simulink model "Vbyf_OpenLoop_Frequencycontrol"  (R2023a)
settings: Solver=FixedStepAuto  StartTime=0.0  StopTime=10.0  FixedStep=1e-6  RelTol=1e-3
libraries: spsIGBTDiodeLib x6, spsCurrentMeasurementLib x3, spsAsynchronousMachineSIUnitsLib x1, simulink x1, spsDCVoltageSourceLib x1, sps_lib x1
settings Model: Creator=hsriv  LastModifiedBy=hsriv

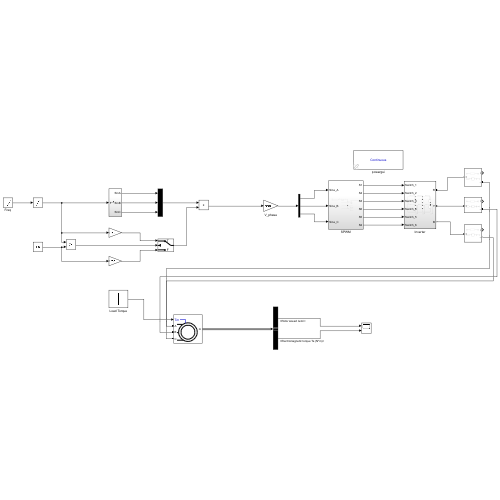
[thumbnail: Simulink's stored preview of the top-level diagram]
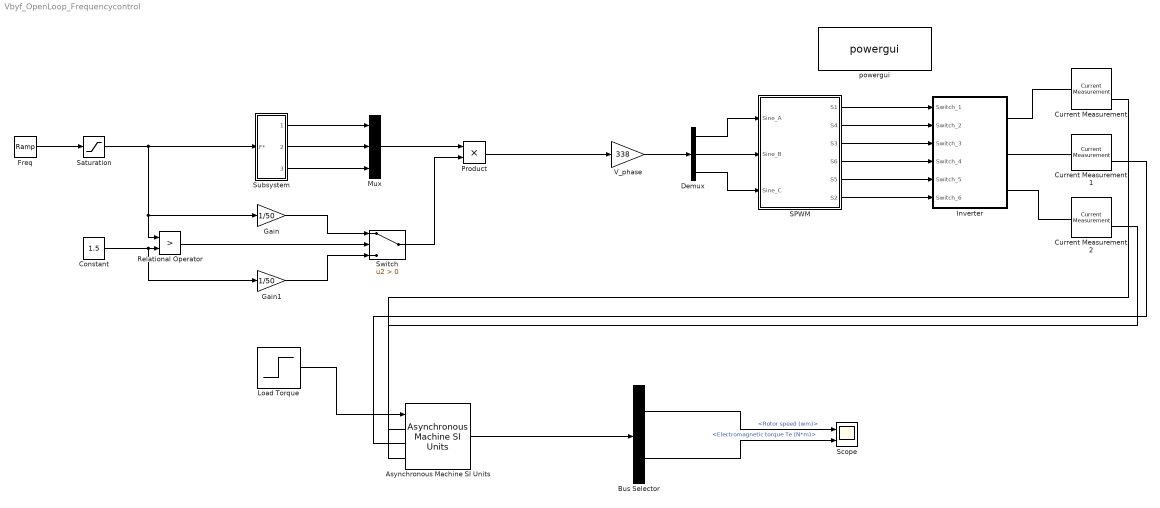
== system Vbyf_OpenLoop_Frequencycontrol ==
  Asynchronous Machine SI Units : spsAsynchronousMachineSIUnitsLib/Asynchronous Machine SI Units  RotorType=Squirrel-cage  PresetModel=No  MechanicalLoad=Torque Tm  ShowDetailedParameters=on  ReferenceFrame=Rotor  Units=SI  MeasurementBus=off  NominalParameters=[1.845e+04 415 50]  VoltageRatio=1  Stator=[0.5968 0.0003495]  Rotor=[0.6258 0.005473]  Cage1=[0.4155 0.002066]  Cage2=[0.4168 0.0003495]  Lm=0.0354  Mechanical=[0.05 0.005879 2]  PolePairs=2  InitialConditions=[1 0 0 0 0 0 0 0]  SimulateSaturation=off  Saturation=[14.03593122, 27.81365428, 53.79336849, 72.68890987, 97.98006896, 148.6815601, 215.7428561, 302.9841135, 428.7778367 ; 230, 322, 414, 460, 506, 552, 598, 644, 690]  LoadFlowParameters=1492000  TsPowergui=0  TsBlock=-1  IterativeModel=Trapezoidal non iterative  IterativeDiscreteModel=Trapezoidal non iterative  Pmec=1.492e+006
  Bus Selector : BusSelector  OutputSignals=Mechanical.Rotor speed (wm),Mechanical.Electromagnetic torque Te (N*m)
  Constant : Constant  Value=1.5
  Current Measurement : spsCurrentMeasurementLib/Current Measurement  PhasorSimulation=off  OutputType=Complex  PSBequivalent=0
  Current Measurement1 : spsCurrentMeasurementLib/Current Measurement  PhasorSimulation=off  OutputType=Complex  PSBequivalent=0
  Current Measurement2 : spsCurrentMeasurementLib/Current Measurement  PhasorSimulation=off  OutputType=Complex  PSBequivalent=0
  Demux : Demux  Outputs=3
  Freq : simulink/Sources/Ramp  slope=100  start=0  InitialOutput=0
  Gain : Gain  Gain=1/50
  Gain1 : Gain  Gain=1/50
  Inverter : Subsystem
  Load Torque : Step  Time=10  Before=0.00001  SampleTime=0
  Mux : Mux  Inputs=3
  Product : Product
  Relational Operator : RelationalOperator  Operator=>  OutDataTypeStr=boolean  RndMeth=Simplest  InputSameDT=off
  SPWM : Subsystem
  Saturation : Saturate  UpperLimit=50  LowerLimit=0
  Scope : Scope  NumInputPorts=2
  Subsystem : Subsystem
  Switch : Switch  Criteria=u2 > Threshold  SaturateOnIntegerOverflow=off  InputSameDT=off
  V_phase : Gain  Gain=338
  powergui : sps_lib/powergui  Priority=1  SimulationMode=Continuous  SampleTime=50e-6  frequency=60  Iterations=50  frequencyindice=50  Pbase=100e6  ErrMax=1e-4  UnitsV=kV  UnitsW=MW  buscounter=0  FunctionMessages=off  echomessages=off  EnableUseOfTLC=off  CurrentSourceSwitches=off  DisableSnubberDevices=off  DisableRonSwitches=off  DisableVfSwitches=off  DisplayEquations=off  AutomaticDiscreteSolvers=off  SolverType=Tustin/Backward Euler (TBE)  Interpol=off  ExternalGateDelay=off  methode=off  Ts=100  x0status=blocks  SPID=on  SwTol=0  HookPort=off  NonlinearTolerance=1e-4  nMaxIteration=100  ContinueOnMaxIteration=off  RestoreLinks=warning  ResistiveCurrentMeasurement=off  Frange=[0:2:500]  Ylog=off  Xlog=on  ShowGrid=off  save=off  variable=ZData  structure=0  ZoomFFT=off  StartTime=0.0  cycles=1  DisplayStyle=1  fundamental=60  FreqAxis=off  MaxFrequency=1000  frequencyindicesteady=1  RmsSteady=1  display=off
  wires:
  Subsystem/1(SinA) -> Mux/1
  Saturation/1 -> Subsystem/1(F*), Gain/1, Relational Operator/1
  Gain/1 -> Switch/1
  Constant/1 -> Gain1/1, Relational Operator/2
  Subsystem/3(SinC) -> Mux/3
  Switch/1 -> Product/2
  Mux/1 -> Product/1
  Freq/1 -> Saturation/1
  Subsystem/2(SinB) -> Mux/2
  Gain1/1 -> Switch/3
  Relational Operator/1 -> Switch/2
  Product/1 -> V_phase/1
  V_phase/1 -> Demux/1
  Demux/2 -> SPWM/2(Sine_B)
  Demux/1 -> SPWM/1(Sine_A)
  Demux/3 -> SPWM/3(Sine_C)
  SPWM/1(S1) -> Inverter/1(Switch_1)
  SPWM/2(S4) -> Inverter/2(Switch_2)
  SPWM/3(S3) -> Inverter/3(Switch_3)
  SPWM/4(S6) -> Inverter/4(Switch_4)
  SPWM/5(S5) -> Inverter/5(Switch_5)
  SPWM/6(S2) -> Inverter/6(Switch_6)
  Asynchronous Machine SI Units/1 -> Bus Selector/1
  Load Torque/1 -> Asynchronous Machine SI Units/1
  Bus Selector/1 -> Scope/1  "<Rotor speed (wm)>"
  Bus Selector/2 -> Scope/2  "<Electromagnetic torque Te (N*m)>"
  connections:
  Inverter/RConn1 -- Current Measurement/LConn1
  Inverter/RConn2 -- Current Measurement1/LConn1
  Inverter/RConn3 -- Current Measurement2/LConn1
  Current Measurement/RConn1 -- Asynchronous Machine SI Units/LConn1
  Current Measurement1/RConn1 -- Asynchronous Machine SI Units/LConn2
  Asynchronous Machine SI Units/LConn3 -- Current Measurement2/RConn1

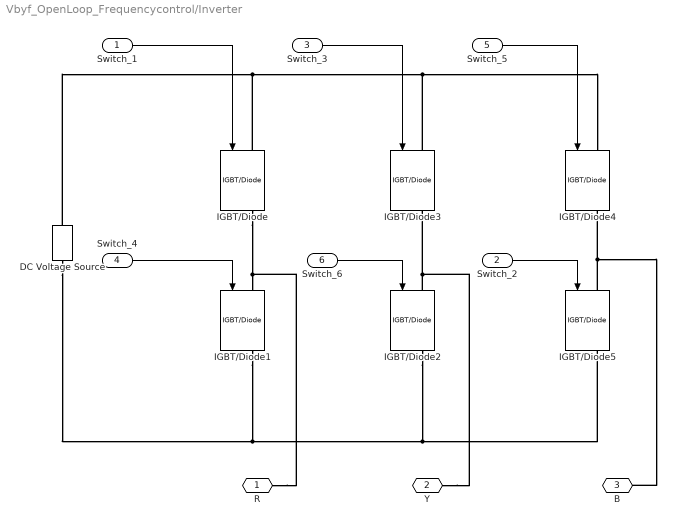
== system Vbyf_OpenLoop_Frequencycontrol/Inverter ==
  Switch_1 : Inport
  Switch_2 : Inport  Port=2
  Switch_3 : Inport  Port=3
  Switch_4 : Inport  Port=4
  Switch_5 : Inport  Port=5
  Switch_6 : Inport  Port=6
  DC Voltage Source : spsDCVoltageSourceLib/DC Voltage Source  Amplitude=700  Measurements=None
  IGBT/Diode{,1..5} (6 alike) : spsIGBTDiodeLib/IGBT//Diode  Ron=1e-3  Rs=1e5  Cs=inf  Measurements=on
  R : PMIOPort  Side=Right
  Y : PMIOPort  Port=2  Side=Right
  B : PMIOPort  Port=3  Side=Right
  wires:
  Switch_3/1 -> IGBT/Diode3/1
  Switch_6/1 -> IGBT/Diode2/1
  Switch_5/1 -> IGBT/Diode4/1
  Switch_4/1 -> IGBT/Diode1/1
  Switch_1/1 -> IGBT/Diode/1
  Switch_2/1 -> IGBT/Diode5/1
  connections:
  DC Voltage Source/LConn1 -- IGBT/Diode1/RConn1 -- IGBT/Diode5/RConn1 -- IGBT/Diode2/RConn1
  IGBT/Diode2/LConn1 -- IGBT/Diode3/RConn1 -- Y/RConn1
  DC Voltage Source/RConn1 -- IGBT/Diode3/LConn1 -- IGBT/Diode4/LConn1 -- IGBT/Diode/LConn1
  IGBT/Diode5/LConn1 -- B/RConn1 -- IGBT/Diode4/RConn1
  IGBT/Diode/RConn1 -- R/RConn1 -- IGBT/Diode1/LConn1

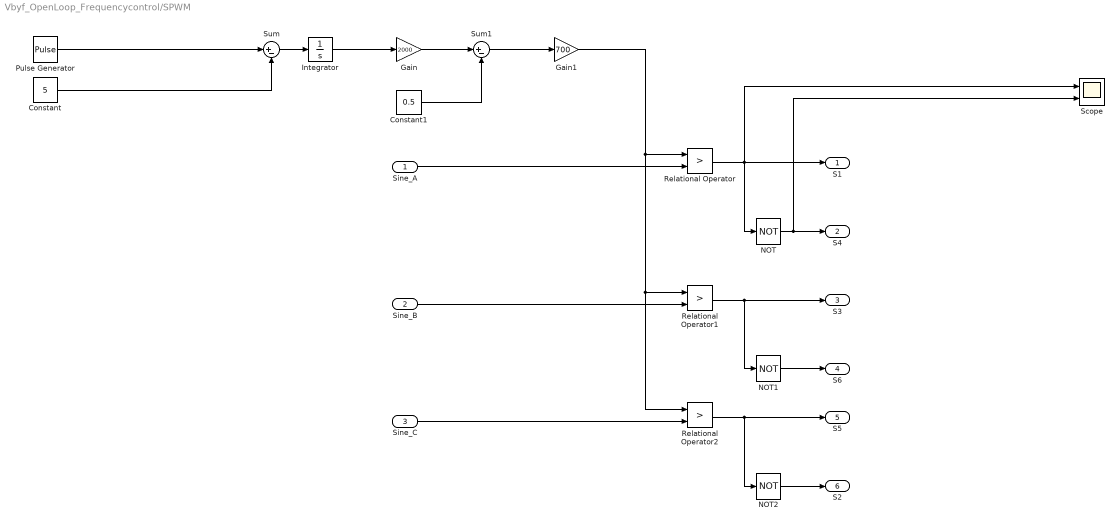
== system Vbyf_OpenLoop_Frequencycontrol/SPWM ==
  Sine_A : Inport
  Sine_B : Inport  Port=2
  Sine_C : Inport  Port=3
  Constant : Constant  Value=5
  Constant1 : Constant  Value=0.5
  Gain : Gain  Gain=2000
  Gain1 : Gain  Gain=700
  Integrator : Integrator
  NOT : Logic  Operator=NOT  IconShape=distinctive  AllPortsSameDT=off  OutDataTypeStr=boolean
  NOT1 : Logic  Operator=NOT  IconShape=distinctive  AllPortsSameDT=off  OutDataTypeStr=boolean
  NOT2 : Logic  Operator=NOT  IconShape=distinctive  AllPortsSameDT=off  OutDataTypeStr=boolean
  Pulse Generator : DiscretePulseGenerator  PulseType=Time based  Amplitude=10  Period=2e-4  PulseWidth=50
  Relational Operator : RelationalOperator  Operator=>  OutDataTypeStr=boolean  RndMeth=Simplest  InputSameDT=off
  Relational Operator1 : RelationalOperator  Operator=>  OutDataTypeStr=boolean  RndMeth=Simplest  InputSameDT=off
  Relational Operator2 : RelationalOperator  Operator=>  OutDataTypeStr=boolean  RndMeth=Simplest  InputSameDT=off
  Scope : Scope  NumInputPorts=2
  Sum : Sum  Inputs=|+-
  Sum1 : Sum  Inputs=|+-
  S1 : Outport
  S4 : Outport  Port=2
  S3 : Outport  Port=3
  S6 : Outport  Port=4
  S5 : Outport  Port=5
  S2 : Outport  Port=6
  wires:
  Constant1/1 -> Sum1/2
  Constant/1 -> Sum/2
  Relational Operator/1 -> S1/1, Scope/1, NOT/1
  Sine_A/1 -> Relational Operator/2
  Sum/1 -> Integrator/1
  Relational Operator2/1 -> S5/1, NOT2/1
  Gain1/1 -> Relational Operator2/1, Relational Operator1/1, Relational Operator/1
  Integrator/1 -> Gain/1
  Relational Operator1/1 -> S3/1, NOT1/1
  Pulse Generator/1 -> Sum/1
  Sum1/1 -> Gain1/1
  Gain/1 -> Sum1/1
  NOT2/1 -> S2/1
  Sine_C/1 -> Relational Operator2/2
  NOT/1 -> S4/1, Scope/2
  NOT1/1 -> S6/1
  Sine_B/1 -> Relational Operator1/2

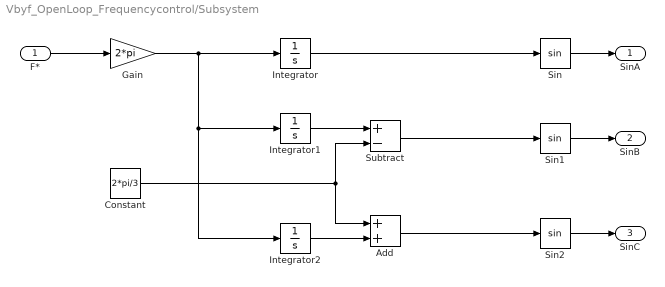
== system Vbyf_OpenLoop_Frequencycontrol/Subsystem ==
  F* : Inport
  Add : Sum
  Constant : Constant  Value=2*pi/3
  Gain : Gain  Gain=2*pi
  Integrator : Integrator
  Integrator1 : Integrator
  Integrator2 : Integrator
  Sin : Trigonometry
  Sin1 : Trigonometry
  Sin2 : Trigonometry
  Subtract : Sum  Inputs=+-
  SinA : Outport
  SinB : Outport  Port=2
  SinC : Outport  Port=3
  wires:
  Gain/1 -> Integrator2/1, Integrator1/1, Integrator/1
  Integrator/1 -> Sin/1
  Sin/1 -> SinA/1
  Integrator1/1 -> Subtract/1
  Subtract/1 -> Sin1/1
  Sin1/1 -> SinB/1
  Integrator2/1 -> Add/2
  Constant/1 -> Subtract/2, Add/1
  Add/1 -> Sin2/1
  Sin2/1 -> SinC/1
  F*/1 -> Gain/1
